simulink model "Prueba_integrador"  (R2017a)
settings: Solver=VariableStepAuto  StartTime=0.0  StopTime=10.0  RelTol=1e-3
libraries: simulink x1
settings Model: Creator=Alfredo Hugueth  LastModifiedBy=Alfredo Hugueth

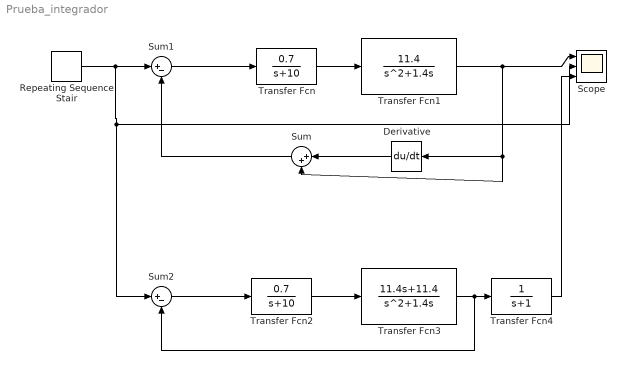
== system Prueba_integrador ==
  Derivative : Derivative  CoefficientInTFapproximation=0
  Repeating Sequence Stair : simulink/Sources/Repeating Sequence Stair  OutValues=[1 0 2 0 1].'  tsamp=1  OutMin=[]  OutMax=[]  OutDataTypeStr=double  OutputDataTypeScalingMode=double  OutDataType=fixdt(0,8)  ConRadixGroup=Best Precision: Vector-wise  OutScaling=2^-12
  Scope : Scope  NumInputPorts=3
  Sum : Sum  Inputs=|++
  Sum1 : Sum  Inputs=|+-
  Sum2 : Sum  Inputs=|+-
  Transfer Fcn : TransferFcn  Numerator=[0.7]  Denominator=[1 10]
  Transfer Fcn1 : TransferFcn  Numerator=[11.4]  Denominator=[1 1.4 0]
  Transfer Fcn2 : TransferFcn  Numerator=[0.7]  Denominator=[1 10]
  Transfer Fcn3 : TransferFcn  Numerator=[11.4 11.4]  Denominator=[1 1.4 0]
  Transfer Fcn4 : TransferFcn  Denominator=[1 1]
  wires:
  Transfer Fcn/1 -> Transfer Fcn1/1
  Transfer Fcn1/1 -> Scope/1, Sum/2, Derivative/1
  Derivative/1 -> Sum/1
  Sum/1 -> Sum1/2
  Repeating Sequence Stair/1 -> Scope/2, Sum2/1, Sum1/1
  Sum1/1 -> Transfer Fcn/1
  Sum2/1 -> Transfer Fcn2/1
  Transfer Fcn2/1 -> Transfer Fcn3/1
  Transfer Fcn3/1 -> Sum2/2, Transfer Fcn4/1
  Transfer Fcn4/1 -> Scope/3
